simulink model "Pendulum_SOFC_integral_oscillator"  (R2022b)
settings: Solver=VariableStepAuto  StartTime=0.0  StopTime=10.0  RelTol=1e-3  EnableMultiTasking=on
values from neighbouring files (symbols this model uses):
  A_osc = [2*cos(w0*Ts)+1, -2*cos(w0*Ts)-1, 1; 1, 0, 0; 0, 1, 0]    [integral_osci_invpendulum_10.m]    (also in integral_osci_invpendulum_100.m; integral_osci_invpendulum_1000.m; integral_osci_pend_1000_personal.m; integral_osci_pend_100_personal.m)
  b = 4.425*1e-6    (= 4.425e-06)    [integral_1000_PJ.m]    (also in integral_100_PJ.m; integral_control_invpendulum_100.m; integral_control_invpendulum_1000.m; integral_control_rotor.m)
  B_osc = [1;0;0]    [integral_osci_invpendulum_10.m]    (also in integral_osci_invpendulum_100.m; integral_osci_invpendulum_1000.m; integral_osci_pend_1000_personal.m; integral_osci_pend_100_personal.m)
  J_pend = J_rotor    (= 1.8053e-05)    [integral_1000_PJ.m]    (also in integral_100_PJ.m; integral_control_invpendulum_100.m; integral_control_invpendulum_1000.m; integral_control_rotor.m)
  K_aug = acker(Aaug,Baug,Pole_SF_int)    [integral_1000_PJ.m]    (also in integral_100_PJ.m; integral_control_invpendulum_100.m = dlqr(Aaug, Baug, 4*[1, 0, 0; 0, 0, 0; 0, 0, 1], 50*1); integral_control_invpendulum_1000.m = dlqr(Aaug, Baug, 2*[1, 0, 0; 0, 0, 0; 0, 0, 1], 50*1); integral_control_rotor_1000.m)
  K_g = m*g*l_c    (= 0.0080536176)    [integral_1000_PJ.m]    (also in integral_100_PJ.m; integral_control_invpendulum_100.m; integral_control_invpendulum_1000.m; integral_control_rotor.m)
  K_int = K_aug(size(A_d,1)+1:size(K_aug,2))    [integral_1000_PJ.m]    (also in integral_100_PJ.m; integral_control_invpendulum_100.m; integral_control_invpendulum_1000.m; integral_control_rotor.m = K_dlqr(size(A_d,1)+1:size(K_aug,2)))
  K_m = 0.025463    [integral_1000_PJ.m]    (also in integral_100_PJ.m; integral_control_invpendulum_100.m; integral_control_invpendulum_1000.m; integral_control_rotor.m)
  K_pend = 0    [integral_1000_PJ.m]    (also in integral_100_PJ.m; integral_control_invpendulum_100.m; integral_control_invpendulum_1000.m; integral_control_rotor.m)
  K_SF = K_aug(1:size(A_d,1))    [integral_1000_PJ.m]    (also in integral_100_PJ.m; integral_control_invpendulum_100.m; integral_control_invpendulum_1000.m; integral_control_rotor.m = K_dlqr(1:size(A_d,1)))
  K_sin = cos(Angle_Pendu)    [integral_1000_PJ.m]    (also in integral_100_PJ.m; integral_control_invpendulum_100.m; integral_control_invpendulum_1000.m; integral_control_rotor.m)
  L_Pred = L_Pred'    [integral_1000_PJ.m]    (also in integral_100_PJ.m; integral_control_invpendulum_100.m; integral_control_invpendulum_1000.m; integral_control_rotor.m = dlqr(A_d', C_d', eye(2), [1]))
  N = 1/freqresp(TF_yrf,[0])    [integral_1000_PJ.m]    (also in integral_100_PJ.m; integral_control_invpendulum_100.m; integral_control_invpendulum_1000.m; integral_control_rotor.m)
  R = 6    [integral_1000_PJ.m]    (also in integral_100_PJ.m; integral_control_invpendulum_100.m; integral_control_invpendulum_1000.m; integral_control_rotor.m)
  saturation = 1.0    (= 1)    [integral_1000_PJ.m]    (also in integral_100_PJ.m; integral_control_invpendulum_100.m; integral_control_invpendulum_1000.m; integral_control_rotor.m)
  Stepsize = 1    [integral_1000_PJ.m]    (also in integral_100_PJ.m; integral_control_invpendulum_100.m; integral_control_invpendulum_1000.m; integral_control_rotor.m)
  Tcomp = 0.0005*Ts*14    (= 7e-06)    [integral_1000_PJ.m]    (also in integral_100_PJ.m = 7e-05; integral_control_invpendulum_100.m = 7e-05; integral_control_invpendulum_1000.m; integral_control_rotor.m)
  Ts = 0.001    [integral_1000_PJ.m]    (also in integral_100_PJ.m = 0.01; integral_control_invpendulum_100.m = 0.01; integral_control_invpendulum_1000.m; integral_control_rotor.m)
  Tss = 1/20000    (= 5e-05)    [integral_1000_PJ.m]    (also in integral_100_PJ.m; integral_control_invpendulum_100.m; integral_control_invpendulum_1000.m; integral_control_rotor.m)
  V_s = 10.5    [integral_1000_PJ.m]    (also in integral_100_PJ.m; integral_control_invpendulum_100.m; integral_control_invpendulum_1000.m; integral_control_rotor.m)
undefined symbols (not defined in the file or in its folder): A_d, B_d, C_d
libraries: spsTriangleGeneratorLib x1, simulink x1
settings Model: Creator=Martin  LastModifiedBy=pruth
settings SolverCC: ZeroCrossControl=DisableAll  ZeroCrossAlgorithm=Adaptive  AlgebraicLoopSolver=TrustRegion
settings DataIOCC: ReturnWorkspaceOutputs=off
settings OptimizationCC: LifeSpan=inf
settings DebuggingCC: MaxConsecutiveZCsMsg=none  UnconnectedInputMsg=warning  UnconnectedOutputMsg=warning  UnconnectedLineMsg=warning  SFUnexpectedBacktrackingDiag=warning  SFNoUnconditionalDefaultTransitionDiag=warning  SFExecutionAtInitializationDiag=none  SFMachineParentedDataDiag=warning  ArithmeticOperatorsInVariantConditions=warning
settings ModelReferenceCC: EnableRefExpFcnMdlSchedulingChecks=on
settings SFSimCC: SimUseLocalCustomCode=off  CustomCodeUndefinedFunction=UseInterfaceOnly
settings RTWCC: RTWUseLocalCustomCode=off  DLArmComputeVersion=19.05
settings CodeAppCC: StateflowObjectComments=on
settings GRTTargetCC: TargetLangStandard=C89/C90 (ANSI)
settings ConfigComp: CovMetricSettings=dw  CovSaveCumulativeToWorkspaceVar=on  CovSaveSingleToWorkspaceVar=on  CovExternalEMLEnable=off

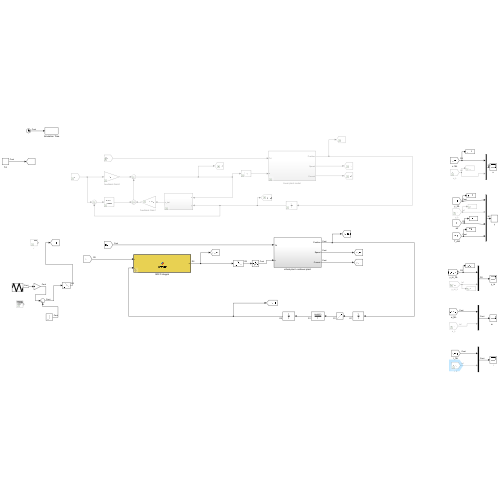
[thumbnail: Simulink's stored preview of the top-level diagram]
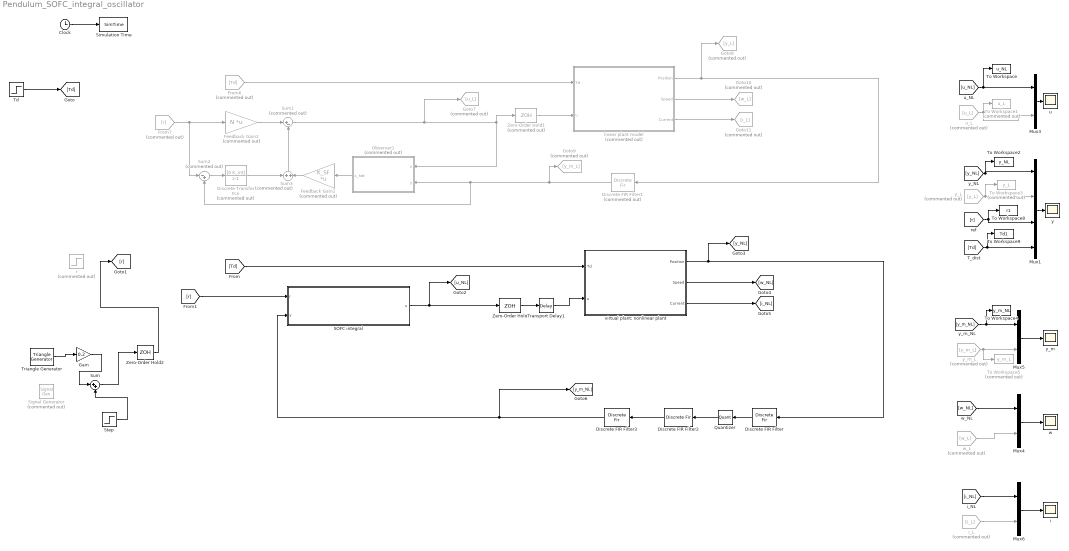
== system Pendulum_SOFC_integral_oscillator ==
  Clock : Clock
  Discrete Transfer Fcn : DiscreteTransferFcn  Commented=on  Numerator=[0 K_int]  Denominator=[1 -1]  SampleTime=Ts
  Discrete FIR Filter : DiscreteFir  Coefficients=[1]  SampleTime=Tss
  Discrete FIR Filter1 : DiscreteFir  Commented=on  Coefficients=[1]  SampleTime=Ts
  Discrete FIR Filter2 : DiscreteFir  Coefficients=[0.25 0.25 0.25 0.25]
  Discrete FIR Filter3 : DiscreteFir  Coefficients=[1]  SampleTime=Ts
  Feedback Gain1 : Gain  Commented=on  Gain=K_SF  Multiplication=Matrix(K*u)
  Feedback Gain2 : Gain  Commented=on  Gain=N  Multiplication=Matrix(K*u)
  From6 : From  Commented=on  GotoTag=Td
  From7 : From  Commented=on  GotoTag=r
  Gain : Gain  Gain=0.2
  Goto10 : Goto  Commented=on  GotoTag=w_L
  Goto11 : Goto  Commented=on  GotoTag=i_L
  Goto7 : Goto  Commented=on  GotoTag=u_L
  Goto8 : Goto  Commented=on  GotoTag=y_L
  Goto9 : Goto  Commented=on  GotoTag=y_m_L
  Mux1 : Mux
  Mux{3..6} (4 alike) : Mux  Inputs=2
  Observer1 : Subsystem  Commented=on
  Quantizer : Quantizer  QuantizationInterval=encoder_resolution
  SOFC integral : MATLAB Function  TreatAsAtomicUnit=on  mask{A=A_d, B=B_d, C=C_d, Aint=A_osc, Bint=B_osc, K=K_aug, L=L_Pred, N=N}
  Signal Generator : SignalGenerator  Commented=on  Amplitude=0.2  Frequency=2
  Simulation Time : ToWorkspace  VariableName=SimTime  SampleTime=-1
  Step : Step  Time=0  After=0.2  SampleTime=0
  Sum : Sum  Inputs=|++
  Sum1 : Sum  Commented=on  Inputs=|+-
  Sum2 : Sum  Commented=on  Inputs=|-+
  Sum3 : Sum  Commented=on  Inputs=+|+
  Td : Step  Time=5  After=0  SampleTime=0
  To Workspace : ToWorkspace  VariableName=u_NL  SampleTime=Ts
  To Workspace1 : ToWorkspace  Commented=on  VariableName=u_L  SampleTime=Ts
  To Workspace2 : ToWorkspace  VariableName=y_NL  SampleTime=Ts
  To Workspace3 : ToWorkspace  Commented=on  VariableName=y_L  SampleTime=Ts
  To Workspace4 : ToWorkspace  VariableName=y_m_NL  SampleTime=Ts
  To Workspace5 : ToWorkspace  Commented=on  VariableName=y_m_L  SampleTime=Ts
  To Workspace8 : ToWorkspace  VariableName=r1  SampleTime=Ts
  To Workspace9 : ToWorkspace  VariableName=Td1  SampleTime=Ts
  Transport Delay1 : TransportDelay  DelayTime=Tcomp  BufferSize=4096  PadeOrder=2
  Triangle Generator : spsTriangleGeneratorLib/Triangle Generator  Freq=1  Phase=90  Ts=0
  Zero-Order Hold : ZeroOrderHold  SampleTime=Ts
  Zero-Order Hold1 : ZeroOrderHold  Commented=on  SampleTime=Ts
  Zero-Order Hold2 : ZeroOrderHold  SampleTime=Ts
  i : Scope
  i_L : From  Commented=on  GotoTag=i_L
  linear plant model : Subsystem  Commented=on
  r : Step  Commented=on  After=Stepsize  SampleTime=Ts
  u : Scope
  u_L : From  Commented=on  GotoTag=u_L
  virtual plant: nonlinear plant : Subsystem
  "w\t" : Scope
  w_L : From  Commented=on  GotoTag=w_L
  y : Scope
  y_L : From  Commented=on  GotoTag=y_L
  y_m : Scope
  y_m_L : From  Commented=on  GotoTag=y_m_L
  wires:
  Clock/1 -> Simulation Time/1
  virtual plant: nonlinear plant/1(Position) -> [y_NL], Discrete FIR Filter/1
  virtual plant: nonlinear plant/2(Speed) -> [w_NL]
  virtual plant: nonlinear plant/3(Current) -> [i_NL]
  Quantizer/1 -> Discrete FIR Filter2/1
  Zero-Order Hold1/1 -> linear plant model/2(u)
  linear plant model/1(Position) -> Goto8/1, Discrete FIR Filter1/1
  Zero-Order Hold/1 -> Transport Delay1/1
  Discrete FIR Filter/1 -> Quantizer/1
  Transport Delay1/1 -> virtual plant: nonlinear plant/2(u)
  [Td] -> virtual plant: nonlinear plant/1(Td)
  From6/1 -> linear plant model/1(Td)
  From7/1 -> Feedback Gain2/1, Sum2/1
  [r] -> SOFC integral/1(r)
  Discrete FIR Filter2/1 -> Discrete FIR Filter3/1
  Sum1/1 -> Goto7/1, Observer1/1(u), Zero-Order Hold1/1
  linear plant model/2(Speed) -> Goto10/1
  linear plant model/3(Current) -> Goto11/1
  Observer1/1(x_hat) -> Feedback Gain1/1
  Feedback Gain2/1 -> Sum1/1
  Discrete FIR Filter3/1 -> SOFC integral/2(y), [y_m_NL]
  SOFC integral/1(u) -> [u_NL], Zero-Order Hold/1
  [u_NL] -> To Workspace/1, Mux3/1
  Mux3/1 -> u/1
  Mux1/1 -> y/1
  [y_NL] -> To Workspace2/1, Mux1/1
  y_L/1 -> To Workspace3/1, Mux1/2
  Mux5/1 -> y_m/1
  [y_m_NL] -> To Workspace4/1, Mux5/1
  y_m_L/1 -> To Workspace5/1, Mux5/2
  Mux4/1 -> "w\t"/1
  [w_NL] -> Mux4/1
  w_L/1 -> Mux4/2
  Mux6/1 -> i/1
  [i_NL] -> Mux6/1
  i_L/1 -> Mux6/2
  u_L/1 -> To Workspace1/1, Mux3/2
  [r] -> To Workspace8/1, Mux1/3
  Td/1 -> [Td]
  Discrete FIR Filter1/1 -> Sum2/2, Observer1/2(y), Goto9/1
  Sum3/1 -> Sum1/2
  Feedback Gain1/1 -> Sum3/2
  [Td] -> To Workspace9/1, Mux1/4
  Discrete Transfer Fcn/1 -> Sum3/1
  Sum2/1 -> Discrete Transfer Fcn/1
  Sum/1 -> Zero-Order Hold2/1
  Zero-Order Hold2/1 -> [r]
  Triangle Generator/1 -> Gain/1
  Step/1 -> Sum/2
  Gain/1 -> Sum/1

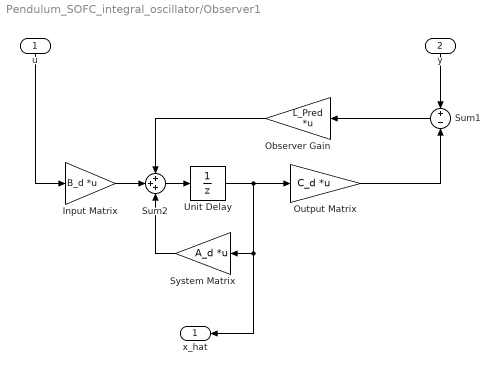
== system Pendulum_SOFC_integral_oscillator/Observer1 ==
  u : Inport
  y : Inport  Port=2
  Input Matrix : Gain  Gain=B_d  Multiplication=Matrix(K*u)
  Observer Gain : Gain  Gain=L_Pred  Multiplication=Matrix(K*u)
  Output Matrix : Gain  Gain=C_d  Multiplication=Matrix(K*u)
  Sum1 : Sum  Inputs=+|-
  Sum2 : Sum  Inputs=+++
  System Matrix : Gain  Gain=A_d  Multiplication=Matrix(K*u)
  Unit Delay : UnitDelay  SampleTime=Ts  HasFrameUpgradeWarning=on
  x_hat : Outport
  wires:
  Sum1/1 -> Observer Gain/1
  System Matrix/1 -> Sum2/3
  Sum2/1 -> Unit Delay/1
  Output Matrix/1 -> Sum1/2
  Input Matrix/1 -> Sum2/2
  Observer Gain/1 -> Sum2/1
  u/1 -> Input Matrix/1
  Unit Delay/1 -> x_hat/1, System Matrix/1, Output Matrix/1
  y/1 -> Sum1/1

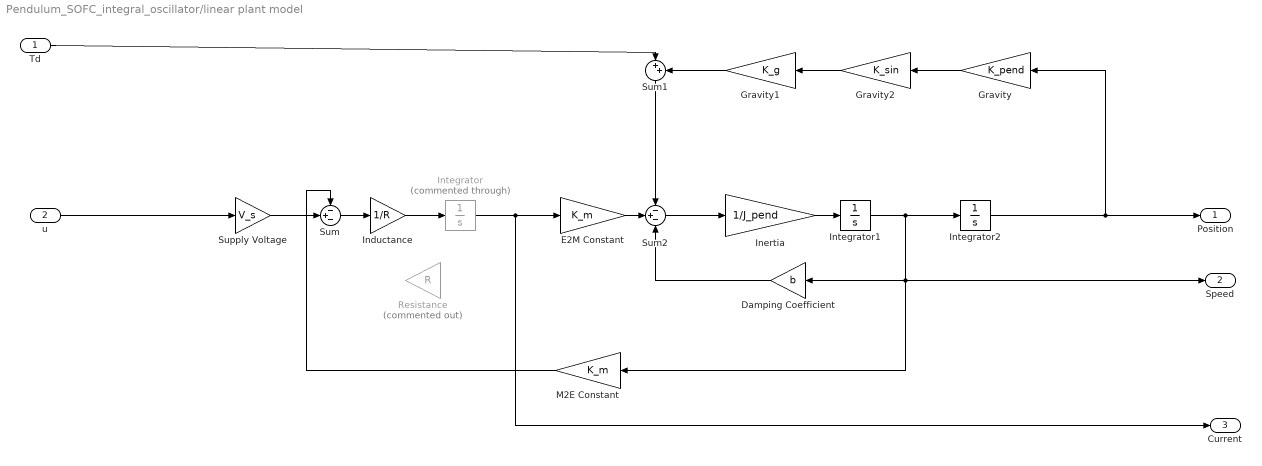
== system Pendulum_SOFC_integral_oscillator/linear plant model ==
  Td : Inport
  u : Inport  Port=2
  Damping Coefficient : Gain  Gain=b
  E2M Constant : Gain  Gain=K_m
  Gravity : Gain  Gain=K_pend
  Gravity1 : Gain  Gain=K_g
  Gravity2 : Gain  Gain=K_sin
  Inductance : Gain  Gain=1/R
  Inertia : Gain  Gain=1/J_pend
  Integrator : Integrator  Commented=through
  Integrator1 : Integrator
  Integrator2 : Integrator
  M2E Constant : Gain  Gain=K_m
  Resistance : Gain  Commented=on  Gain=R
  Sum : Sum  Inputs=-+-
  Sum1 : Sum  Inputs=|++
  Sum2 : Sum  Inputs=-+-
  Supply Voltage : Gain  Gain=V_s
  Position : Outport
  Speed : Outport  Port=2
  Current : Outport  Port=3
  wires:
  Damping Coefficient/1 -> Sum2/3
  Sum1/1 -> Sum2/1
  Gravity/1 -> Gravity2/1
  Integrator/1 -> E2M Constant/1, Current/1
  Integrator1/1 -> Damping Coefficient/1, Speed/1, M2E Constant/1, Integrator2/1
  Sum/1 -> Inductance/1
  Inductance/1 -> Integrator/1
  Supply Voltage/1 -> Sum/2
  M2E Constant/1 -> Sum/1
  Sum2/1 -> Inertia/1
  Inertia/1 -> Integrator1/1
  E2M Constant/1 -> Sum2/2
  u/1 -> Supply Voltage/1
  Td/1 -> Sum1/1
  Integrator2/1 -> Gravity/1, Position/1
  Gravity1/1 -> Sum1/2
  Gravity2/1 -> Gravity1/1

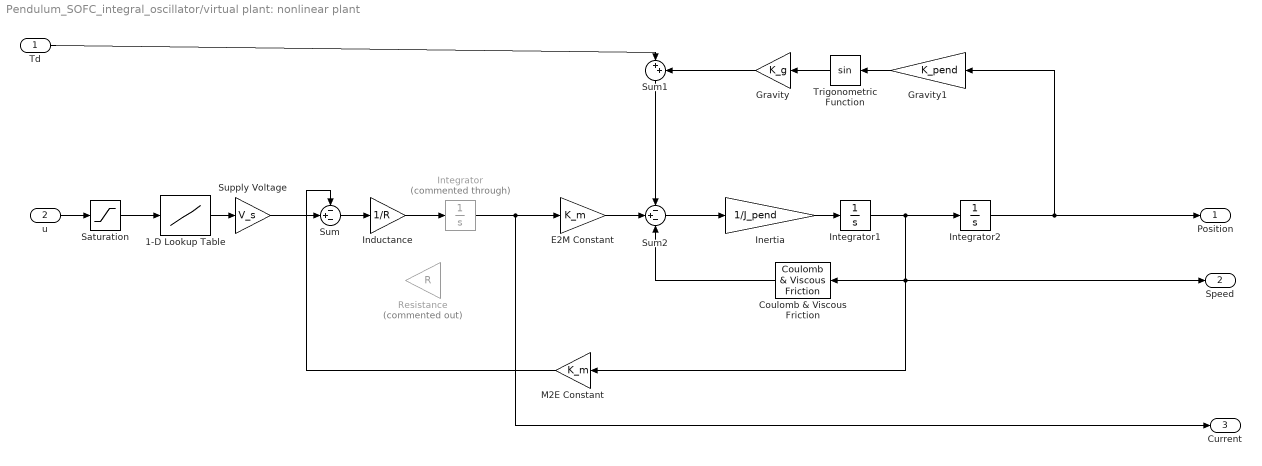
== system Pendulum_SOFC_integral_oscillator/virtual plant: nonlinear plant ==
  Td : Inport
  u : Inport  Port=2
  1-D Lookup Table : Lookup_n-D  NumberOfTableDimensions=1  BreakpointsForDimension1=[-1,1]  Table=[-10.5,10.5]/V_s  InternalRulePriority=Speed  RndMeth=Simplest
  Coulomb & Viscous Friction : simulink/Discontinuities/Coulomb & Viscous Friction  offset=Friction_static  gain=b
  E2M Constant : Gain  Gain=K_m
  Gravity : Gain  Gain=K_g
  Gravity1 : Gain  Gain=K_pend
  Inductance : Gain  Gain=1/R
  Inertia : Gain  Gain=1/J_pend
  Integrator : Integrator  Commented=through
  Integrator1 : Integrator
  Integrator2 : Integrator
  M2E Constant : Gain  Gain=K_m
  Resistance : Gain  Commented=on  Gain=R
  Saturation : Saturate  UpperLimit=saturation  LowerLimit=-saturation
  Sum : Sum  Inputs=-+-
  Sum1 : Sum  Inputs=|++
  Sum2 : Sum  Inputs=-+-
  Supply Voltage : Gain  Gain=V_s
  Trigonometric Function : Trigonometry
  Position : Outport
  Speed : Outport  Port=2
  Current : Outport  Port=3
  wires:
  Coulomb & Viscous Friction/1 -> Sum2/3
  Gravity/1 -> Sum1/2
  Integrator/1 -> E2M Constant/1, Current/1
  Integrator1/1 -> Coulomb & Viscous Friction/1, Speed/1, M2E Constant/1, Integrator2/1
  Trigonometric Function/1 -> Gravity/1
  Sum/1 -> Inductance/1
  Inductance/1 -> Integrator/1
  Supply Voltage/1 -> Sum/2
  M2E Constant/1 -> Sum/1
  Sum2/1 -> Inertia/1
  Inertia/1 -> Integrator1/1
  Saturation/1 -> 1-D Lookup Table/1
  u/1 -> Saturation/1
  E2M Constant/1 -> Sum2/2
  Integrator2/1 -> Position/1, Gravity1/1
  1-D Lookup Table/1 -> Supply Voltage/1
  Td/1 -> Sum1/1
  Gravity1/1 -> Trigonometric Function/1
  Sum1/1 -> Sum2/1

== matlab function Pendulum_SOFC_integral_oscillator/SOFC integral ==
  data: r input; u output; y input; A parameter; B parameter; C parameter; K parameter; L parameter; N parameter; Aint parameter; Bint parameter
function u = controller(r,y,A, B, C, K, L, N, Aint, Bint)

persistent xhat xint;  %memory for the state

  if isempty(xhat)  %local variable initialization
      n=size(L,1);
        xhat=zeros(n,1); 
      m = size(K,2)-n;
        xint=zeros(m,1);  
  end
xaug=[xhat; xint]; %Augmented state include the state for the integrator
%u = -K*xaug+N*r; %Control computation with integral action 
u_unsat = -K*xaug+N*r; %Control computation with integral action 
u= sign(u_unsat)*min(1,abs(u_unsat));
%DAC(u) send out control here to minimize computation delay
%Update the next state next
xhat = (A-L*C)*xhat + B*u + L*y;
xint = Aint*xint + Bint*(y-r);
